simulink library "powerlib"  (Simulink 6.0)
settings: Solver=ode45  SolverMode=SingleTasking  StartTime=0.0  StopTime=10.0  RelTol=1e-3
undefined symbols (not defined in the file or in its folder): com, ctrl1, Da, DiscIntNeverNeededParam, dtha, etat, FA, find_system, Ha, j, Ka, Ki, Kv, q0, Rground, sel, st_a, st_b, st_c, sta, stb, stc, T1, T2, T3, T4
libraries: powerlib_models x30, powerlib x25, simulink_extras x6, powerlib_extras x3, simulink x2
(part 7 of 7)

== system powerlib/Phasor Elements/Static Var Compensator/I1 Time delay  Td ==
  I1 cmplx : Inport  Orientation=left  Port=1  LatchInput=off
  Complex to Real-Imag : ComplexToRealImag  Orientation=left
  Real-Imag to Complex : RealImagToComplex  Orientation=left
  Transport Delay1 : TransportDelay  Orientation=left  DelayTime=Td
  Transport Delay2 : TransportDelay  Orientation=left  DelayTime=Td
  Out1 : Outport  Orientation=left
  wires:
  I1 cmplx/1 -> Complex to Real-Imag/1
  Real-Imag to Complex/1 -> Out1/1
  Complex to Real-Imag/1 -> Transport Delay1/1
  Complex to Real-Imag/2 -> Transport Delay2/1
  Transport Delay1/1 -> Real-Imag to Complex/1
  Transport Delay2/1 -> Real-Imag to Complex/2

== system powerlib/Phasor Elements/Static Var Compensator/I2 Time delay I2 ==
  I1 cmplx : Inport  Orientation=left  Port=1  LatchInput=off
  Complex to Real-Imag : ComplexToRealImag  Orientation=left
  Real-Imag to Complex : RealImagToComplex  Orientation=left
  Transport Delay1 : TransportDelay  Orientation=left  DelayTime=Td
  Transport Delay2 : TransportDelay  Orientation=left  DelayTime=Td
  Out1 : Outport  Orientation=left
  wires:
  Transport Delay2/1 -> Real-Imag to Complex/2
  Transport Delay1/1 -> Real-Imag to Complex/1
  Complex to Real-Imag/2 -> Transport Delay2/1
  Complex to Real-Imag/1 -> Transport Delay1/1
  Real-Imag to Complex/1 -> Out1/1
  I1 cmplx/1 -> Complex to Real-Imag/1

== system powerlib/Phasor Elements/Static Var Compensator/Phasors-->V1 V2 ==
  Vab Vbc cmplx : Inport  Port=1  LatchInput=off
  (a^2)/3 : Gain  Gain=1/3*exp(-j*2*pi/3)  SaturateOnIntegerOverflow=on
  Demux : Demux  Outputs=2
  Gain : Gain  Gain=1/3  SaturateOnIntegerOverflow=on
  Gain1 : Gain  Gain=1/3  SaturateOnIntegerOverflow=on
  Sum3 : Sum  Inputs=+-  SaturateOnIntegerOverflow=on  InputSameDT=on
  Sum4 : Sum  Inputs=+-  SaturateOnIntegerOverflow=on  InputSameDT=on
  V>pu : Gain  Gain=1/Vbase  SaturateOnIntegerOverflow=on
  a/3 : Gain  Gain=1/3*exp(j*2*pi/3)  SaturateOnIntegerOverflow=on
  V1_pu : Outport
  V2_pu : Outport  Port=2
  wires:
  Sum4/1 -> V2_pu/1  "V2"
  (a^2)/3/1 -> Sum3/2
  Demux/2 -> (a^2)/3/1, a/3/1
  Gain/1 -> Sum3/1
  Vab Vbc cmplx/1 -> V>pu/1
  Gain1/1 -> Sum4/1
  a/3/1 -> Sum4/2
  Demux/1 -> Gain/1, Gain1/1
  Sum3/1 -> V1_pu/1  "V1"
  V>pu/1 -> Demux/1

== system powerlib/Phasor Elements/Static Var Compensator/Voltage regulator ==
  V1meas (pu) : Inport  Port=1  LatchInput=off
  Vref (pu) : Inport  Port=2  LatchInput=off
  Break algebraic loop : TransferFcn  Orientation=left  Denominator=[100e-6 1]
  Droop : Gain  Orientation=left  Gain=Xs  SaturateOnIntegerOverflow=on
  Integrator : Integrator  LimitOutput=on  UpperSaturationLimit=Bmax  LowerSaturationLimit=Bmin
  Ki : Gain  Gain=Ki  SaturateOnIntegerOverflow=on
  Kp : Gain  Gain=Kp  SaturateOnIntegerOverflow=on
  Product : Product  Orientation=down  SaturateOnIntegerOverflow=on  InputSameDT=on
  Saturation : Saturate  UpperLimit=Bmax  LowerLimit=Bmin
  Sum : Sum  Inputs=-+-  SaturateOnIntegerOverflow=on  InputSameDT=on
  Sum1 : Sum  SaturateOnIntegerOverflow=on
  B (pu) : Outport  InitialOutput=0
  wires:
  Sum1/1 -> Product/2, B (pu)/1
  Saturation/1 -> Sum1/1
  Integrator/1 -> Sum1/2
  Kp/1 -> Saturation/1
  Product/1 -> Break algebraic loop/1
  Sum/1 -> Kp/1, Ki/1
  Vref (pu)/1 -> Sum/2
  Ki/1 -> Integrator/1
  V1meas (pu)/1 -> Sum/1, Product/1
  Droop/1 -> Sum/3
  Break algebraic loop/1 -> Droop/1

== system powerlib/Power Electronics/Detailed Thyristor/Measurement list ==
  In1 : Inport  Port=1  LatchInput=off
  Bus Creator1 : BusCreator  DialogController=Simulink.DDGSource_Bus  Inputs=2
  Demux : Demux  Outputs=[1,1]
  Out1 : Outport
  wires:
  Demux/2 -> Bus Creator1/2  "Thyristor voltage"
  Demux/1 -> Bus Creator1/1  "Thyristor current"
  Bus Creator1/1 -> Out1/1
  In1/1 -> Demux/1

== system powerlib/Power Electronics/Diode/Measurement list ==
  In1 : Inport  Port=1  LatchInput=off
  Bus Creator1 : BusCreator  DialogController=Simulink.DDGSource_Bus  Inputs=2
  Demux : Demux  Outputs=[1,1]
  Out1 : Outport
  wires:
  In1/1 -> Demux/1
  Bus Creator1/1 -> Out1/1
  Demux/1 -> Bus Creator1/1  "Diode current"
  Demux/2 -> Bus Creator1/2  "Diode voltage"

== system powerlib/Power Electronics/Gto/Measurement list ==
  In1 : Inport  Port=1  LatchInput=off
  Bus Creator1 : BusCreator  DialogController=Simulink.DDGSource_Bus  Inputs=2
  Demux : Demux  Outputs=[1,1]
  Out1 : Outport
  wires:
  Demux/2 -> Bus Creator1/2  "GTO voltage"
  Demux/1 -> Bus Creator1/1  "GTO current"
  Bus Creator1/1 -> Out1/1
  In1/1 -> Demux/1

== system powerlib/Power Electronics/IGBT/Measurement list ==
  In1 : Inport  Port=1  LatchInput=off
  Bus Creator1 : BusCreator  DialogController=Simulink.DDGSource_Bus  Inputs=2
  Demux : Demux  Outputs=[1,1]
  Out1 : Outport
  wires:
  Demux/2 -> Bus Creator1/2  "IGBT voltage"
  Demux/1 -> Bus Creator1/1  "IGBT current"
  Bus Creator1/1 -> Out1/1
  In1/1 -> Demux/1

== system powerlib/Power Electronics/Ideal Switch/Measurement list ==
  In1 : Inport  Port=1  LatchInput=off
  Bus Creator1 : BusCreator  DialogController=Simulink.DDGSource_Bus  Inputs=2
  Demux : Demux  Outputs=[1,1]
  Out1 : Outport
  wires:
  In1/1 -> Demux/1
  Bus Creator1/1 -> Out1/1
  Demux/1 -> Bus Creator1/1  "Switch current"
  Demux/2 -> Bus Creator1/2  "Switch voltage"

== system powerlib/Power Electronics/Mosfet/Measurement list ==
  In1 : Inport  Port=1  LatchInput=off
  Bus Creator1 : BusCreator  DialogController=Simulink.DDGSource_Bus  Inputs=2
  Demux : Demux  Outputs=[1,1]
  Out1 : Outport
  wires:
  In1/1 -> Demux/1
  Bus Creator1/1 -> Out1/1
  Demux/1 -> Bus Creator1/1  "Mosfet current"
  Demux/2 -> Bus Creator1/2  "Mosfet voltage"

== system powerlib/Power Electronics/Thyristor/Measurement list ==
  In1 : Inport  Port=1  LatchInput=off
  Bus Creator1 : BusCreator  DialogController=Simulink.DDGSource_Bus  Inputs=2
  Demux : Demux  Outputs=[1,1]
  Out1 : Outport
  wires:
  In1/1 -> Demux/1
  Bus Creator1/1 -> Out1/1
  Demux/1 -> Bus Creator1/1  "Thyristor current"
  Demux/2 -> Bus Creator1/2  "Thyristor voltage"

== system powerlib/Machines/Steam Turbine and Governor/4 mass shaft/1 mass ==
  Tt_1-4 : Inport  Port=1  LatchInput=off
  dth_gen : Inport  Port=2  LatchInput=off
  Enable : EnablePort
  Ground : Ground
  Ground1 : Ground  Orientation=left
  Mass2 : Subsystem  mask(Generic rotating mass){H=Ha(1), K=Ka(1), D=Da(1), dth0=dtha(1)}
      mask prompts: H "Inertia H (p.u.)"; K "Rigidity K (p.u.):"; D "Damping D (p.u.):"; dth0 "Initial angle deviation delta_theta (rad):"
  Mux : Mux  Inputs=[3 1]
  Mux1 : Mux  Inputs=[3 1]
  Selector : Selector  Elements=sel{1}  InputPortWidth=4
  Terminator : Terminator
  Ts_5-2 : Outport  InitialOutput=[0,0,0,0]
  dw_5-2 : Outport  Port=2  InitialOutput=[0,0,0,0]
  Tm_gen : Outport  Port=3
  wires:
  Mass2/2(Ts_k) -> Tm_gen/1, Mux/2
  dth_gen/1 -> Mass2/3(deltat_k-1)
  Mass2/1(deltat_k) -> Terminator/1
  Ground/1 -> Mass2/1(Ts_k+1)
  Selector/1 -> Mass2/2(Tt_k)
  Mux/1 -> Ts_5-2/1
  Tt_1-4/1 -> Selector/1
  Ground1/1 -> Mux/1, Mux1/1
  Mass2/3(dw) -> Mux1/2
  Mux1/1 -> dw_5-2/1

== system powerlib/Machines/Steam Turbine and Governor/4 mass shaft/2 masses ==
  Tt_1-4 : Inport  Port=1  LatchInput=off
  dth_gen : Inport  Port=2  LatchInput=off
  Enable : EnablePort
  Demux : Demux  Outputs=2
  Ground : Ground
  Ground1 : Ground  Orientation=left
  Mass2 : Subsystem  mask(Generic rotating mass){H=Ha(1), K=Ka(1), D=Da(1), dth0=dtha(1)}
      mask prompts: H "Inertia H (p.u.)"; K "Rigidity K (p.u.):"; D "Damping D (p.u.):"; dth0 "Initial angle deviation delta_theta (rad):"
  Mass3 : Subsystem  mask(Generic rotating mass){H=Ha(2), K=Ka(2), D=Da(2), dth0=dtha(2)}
      mask prompts: H "Inertia H (p.u.)"; K "Rigidity K (p.u.):"; D "Damping D (p.u.):"; dth0 "Initial angle deviation delta_theta (rad):"
  Mux : Mux  Inputs=[ 2 1 1 ]
  Mux1 : Mux  Inputs=[ 2 1 1 ]
  Selector : Selector  Elements=sel{2}  InputPortWidth=4
  Terminator : Terminator
  Ts_5-2 : Outport  InitialOutput=[0,0,0,0]
  dw_5-2 : Outport  Port=2  InitialOutput=[0,0,0,0]
  Tm_gen : Outport  Port=3
  wires:
  Mass2/2(Ts_k) -> Tm_gen/1, Mux/3
  dth_gen/1 -> Mass2/3(deltat_k-1)
  Mass2/1(deltat_k) -> Mass3/3(deltat_k-1)
  Demux/2 -> Mass2/2(Tt_k)
  Ground/1 -> Mass3/1(Ts_k+1)
  Mass3/1(deltat_k) -> Terminator/1
  Mass3/2(Ts_k) -> Mass2/1(Ts_k+1), Mux/2
  Mux/1 -> Ts_5-2/1
  Selector/1 -> Demux/1
  Tt_1-4/1 -> Selector/1
  Demux/1 -> Mass3/2(Tt_k)
  Ground1/1 -> Mux/1, Mux1/1
  Mux1/1 -> dw_5-2/1
  Mass3/3(dw) -> Mux1/2
  Mass2/3(dw) -> Mux1/3

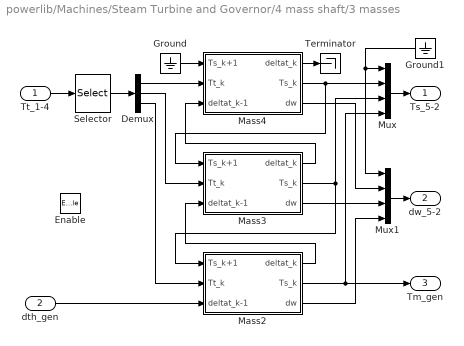
== system powerlib/Machines/Steam Turbine and Governor/4 mass shaft/3 masses ==
  Tt_1-4 : Inport  Port=1  LatchInput=off
  dth_gen : Inport  Port=2  LatchInput=off
  Enable : EnablePort
  Demux : Demux  Outputs=3
  Ground : Ground
  Ground1 : Ground  Orientation=left
  Mass2 : Subsystem  mask(Generic rotating mass){H=Ha(1), K=Ka(1), D=Da(1), dth0=dtha(1)}
      mask prompts: H "Inertia H (p.u.)"; K "Rigidity K (p.u.):"; D "Damping D (p.u.):"; dth0 "Initial angle deviation delta_theta (rad):"
  Mass3 : Subsystem  mask(Generic rotating mass){H=Ha(2), K=Ka(2), D=Da(2), dth0=dtha(2)}
      mask prompts: H "Inertia H (p.u.)"; K "Rigidity K (p.u.):"; D "Damping D (p.u.):"; dth0 "Initial angle deviation delta_theta (rad):"
  Mass4 : Subsystem  mask(Generic rotating mass){H=Ha(3), K=Ka(3), D=Da(3), dth0=dtha(3)}
      mask prompts: H "Inertia H (p.u.)"; K "Rigidity K (p.u.):"; D "Damping D (p.u.):"; dth0 "Initial angle deviation delta_theta (rad):"
  Mux : Mux
  Mux1 : Mux
  Selector : Selector  Elements=sel{3}  InputPortWidth=4
  Terminator : Terminator
  Ts_5-2 : Outport  InitialOutput=[0,0,0,0]
  dw_5-2 : Outport  Port=2  InitialOutput=[0,0,0,0]
  Tm_gen : Outport  Port=3
  wires:
  Mass3/2(Ts_k) -> Mass2/1(Ts_k+1), Mux/3
  Tt_1-4/1 -> Selector/1
  Selector/1 -> Demux/1
  Mass2/2(Ts_k) -> Mux/4, Tm_gen/1
  dth_gen/1 -> Mass2/3(deltat_k-1)
  Mass4/1(deltat_k) -> Terminator/1
  Ground/1 -> Mass4/1(Ts_k+1)
  Demux/1 -> Mass4/2(Tt_k)
  Demux/2 -> Mass3/2(Tt_k)
  Demux/3 -> Mass2/2(Tt_k)
  Mass2/1(deltat_k) -> Mass3/3(deltat_k-1)
  Mass3/1(deltat_k) -> Mass4/3(deltat_k-1)
  Mass4/2(Ts_k) -> Mass3/1(Ts_k+1), Mux/2
  Mass4/3(dw) -> Mux1/2
  Mass3/3(dw) -> Mux1/3
  Mux/1 -> Ts_5-2/1
  Ground1/1 -> Mux/1, Mux1/1
  Mux1/1 -> dw_5-2/1
  Mass2/3(dw) -> Mux1/4

== system powerlib/Machines/Steam Turbine and Governor/4 mass shaft/4 masses ==
  Tt_1-4 : Inport  Port=1  LatchInput=off
  dth_gen : Inport  Port=2  LatchInput=off
  Enable : EnablePort
  Demux : Demux
  Ground : Ground
  Mass2 : Subsystem  mask(Generic rotating mass){H=Ha(1), K=Ka(1), D=Da(1), dth0=dtha(1)}
      mask prompts: H "Inertia H (p.u.)"; K "Rigidity K (p.u.):"; D "Damping D (p.u.):"; dth0 "Initial angle deviation delta_theta (rad):"
  Mass3 : Subsystem  mask(Generic rotating mass){H=Ha(2), K=Ka(2), D=Da(2), dth0=dtha(2)}
      mask prompts: H "Inertia H (p.u.)"; K "Rigidity K (p.u.):"; D "Damping D (p.u.):"; dth0 "Initial angle deviation delta_theta (rad):"
  Mass4 : Subsystem  mask(Generic rotating mass){H=Ha(3), K=Ka(3), D=Da(3), dth0=dtha(3)}
      mask prompts: H "Inertia H (p.u.)"; K "Rigidity K (p.u.):"; D "Damping D (p.u.):"; dth0 "Initial angle deviation delta_theta (rad):"
  Mass5 : Subsystem  mask(Generic rotating mass){H=Ha(4), K=Ka(4), D=Da(4), dth0=dtha(4)}
      mask prompts: H "Inertia H (p.u.)"; K "Rigidity K (p.u.):"; D "Damping D (p.u.):"; dth0 "Initial angle deviation delta_theta (rad):"
  Mux : Mux
  Mux1 : Mux
  Terminator : Terminator
  Ts_5-2 : Outport  InitialOutput=[0,0,0,0]
  dw_5-2 : Outport  Port=2  InitialOutput=[0,0,0,0]
  Tm_gen : Outport  Port=3
  wires:
  Mass2/2(Ts_k) -> Tm_gen/1, Mux/4
  dth_gen/1 -> Mass2/3(deltat_k-1)
  Tt_1-4/1 -> Demux/1
  Mass3/2(Ts_k) -> Mux/3, Mass2/1(Ts_k+1)
  Mass4/2(Ts_k) -> Mux/2, Mass3/1(Ts_k+1)
  Mass5/2(Ts_k) -> Mass4/1(Ts_k+1), Mux/1
  Mass4/1(deltat_k) -> Mass5/3(deltat_k-1)
  Mass3/1(deltat_k) -> Mass4/3(deltat_k-1)
  Mass2/1(deltat_k) -> Mass3/3(deltat_k-1)
  Demux/4 -> Mass2/2(Tt_k)
  Demux/3 -> Mass3/2(Tt_k)
  Demux/2 -> Mass4/2(Tt_k)
  Demux/1 -> Mass5/2(Tt_k)
  Ground/1 -> Mass5/1(Ts_k+1)
  Mass5/1(deltat_k) -> Terminator/1
  Mux/1 -> Ts_5-2/1
  Mass5/3(dw) -> Mux1/1
  Mass4/3(dw) -> Mux1/2
  Mux1/1 -> dw_5-2/1
  Mass3/3(dw) -> Mux1/3
  Mass2/3(dw) -> Mux1/4

== system powerlib/Machines/Steam Turbine and Governor/steam turbine/Stage1 ==
  In1 : Inport  Port=1  LatchInput=off
  Constant1 : Constant  Orientation=down  Value=Ta(4)~=0
  Stage4 : Subsystem  TreatAsAtomicUnit=on
  Switch3 : Switch  Threshold=0.5  InputSameDT=on
  Out1 : Outport
  wires:
  Switch3/1 -> Out1/1
  In1/1 -> Switch3/3, Stage4/1(In1)
  Constant1/1 -> Switch3/2, Stage4/Enable
  Stage4/1(Out1) -> Switch3/1

== system powerlib/Machines/Steam Turbine and Governor/steam turbine/Stage2 ==
  In1 : Inport  Port=1  LatchInput=off
  Constant2 : Constant  Orientation=down  Value=Ta(3)~=0
  Stage3 : Subsystem  TreatAsAtomicUnit=on
  Switch2 : Switch  Threshold=0.5  InputSameDT=on
  Out1 : Outport
  wires:
  In1/1 -> Switch2/3, Stage3/1(In1)
  Switch2/1 -> Out1/1
  Constant2/1 -> Switch2/2, Stage3/Enable
  Stage3/1(Out1) -> Switch2/1

== system powerlib/Machines/Steam Turbine and Governor/steam turbine/Stage3  ==
  In1 : Inport  Port=1  LatchInput=off
  Constant3 : Constant  Orientation=down  Value=Ta(2)~=0
  Stage2 : Subsystem  TreatAsAtomicUnit=on
  Switch1 : Switch  Threshold=0.5  InputSameDT=on
  Out1 : Outport
  wires:
  In1/1 -> Switch1/3, Stage2/1(In1)
  Switch1/1 -> Out1/1
  Constant3/1 -> Switch1/2, Stage2/Enable
  Stage2/1(Out1) -> Switch1/1

== system powerlib/Machines/Steam Turbine and Governor/steam turbine/Stage4 ==
  In1 : Inport  Port=1  LatchInput=off
  Constant4 : Constant  Orientation=down  Value=Ta(1)~=0
  Stage1 : Subsystem  TreatAsAtomicUnit=on
  Switch : Switch  Threshold=0.5  InputSameDT=on
  Out1 : Outport
  wires:
  Switch/1 -> Out1/1
  Stage1/1(Out1) -> Switch/1
  In1/1 -> Switch/3, Stage1/1(In1)
  Constant4/1 -> Switch/2, Stage1/Enable

== system powerlib/Machines/Steam Turbine and Governor/4 mass shaft/1 mass/Mass2 ==
  Ts_k+1 : Inport  Port=1  LatchInput=off
  Tt_k : Inport  Port=2  LatchInput=off
  deltat_k-1 : Inport  Port=3  LatchInput=off
  Gain10 : Gain  Gain=D  SaturateOnIntegerOverflow=on
  Gain11 : Gain  Gain=K  SaturateOnIntegerOverflow=on
  Gain9 : Gain  Gain=1/(2*H)  SaturateOnIntegerOverflow=on
  Integrator6 : Integrator
  Integrator7 : Integrator  InitialCondition=dth0
  Sum11 : Sum  Orientation=left  Inputs=|+-  SaturateOnIntegerOverflow=on  InputSameDT=on
  Sum9 : Sum  Inputs=+|+|-|-  SaturateOnIntegerOverflow=on  InputSameDT=on
  pu2radpersec : Gain  Gain=120*pi  SaturateOnIntegerOverflow=on
  deltat_k : Outport  InitialOutput=0
  Ts_k : Outport  Port=2  InitialOutput=0
  dw : Outport  Port=3  InitialOutput=0
  wires:
  deltat_k-1/1 -> Sum11/2
  Sum11/1 -> Gain11/1
  Integrator7/1 -> deltat_k/1, Sum11/1
  pu2radpersec/1 -> Integrator7/1
  Integrator6/1 -> pu2radpersec/1, Gain10/1, dw/1
  Tt_k/1 -> Sum9/2
  Sum9/1 -> Gain9/1
  Gain10/1 -> Sum9/4
  Gain11/1 -> Ts_k/1, Sum9/3
  Ts_k+1/1 -> Sum9/1
  Gain9/1 -> Integrator6/1

== system powerlib/Machines/Steam Turbine and Governor/4 mass shaft/2 masses/Mass2 ==
  Ts_k+1 : Inport  Port=1  LatchInput=off
  Tt_k : Inport  Port=2  LatchInput=off
  deltat_k-1 : Inport  Port=3  LatchInput=off
  Gain10 : Gain  Gain=D  SaturateOnIntegerOverflow=on
  Gain11 : Gain  Gain=K  SaturateOnIntegerOverflow=on
  Gain9 : Gain  Gain=1/(2*H)  SaturateOnIntegerOverflow=on
  Integrator6 : Integrator
  Integrator7 : Integrator  InitialCondition=dth0
  Sum11 : Sum  Orientation=left  Inputs=|+-  SaturateOnIntegerOverflow=on  InputSameDT=on
  Sum9 : Sum  Inputs=+|+|-|-  SaturateOnIntegerOverflow=on  InputSameDT=on
  pu2radpersec : Gain  Gain=120*pi  SaturateOnIntegerOverflow=on
  deltat_k : Outport  InitialOutput=0
  Ts_k : Outport  Port=2  InitialOutput=0
  dw : Outport  Port=3  InitialOutput=0
  wires:
  deltat_k-1/1 -> Sum11/2
  Sum11/1 -> Gain11/1
  Integrator7/1 -> deltat_k/1, Sum11/1
  pu2radpersec/1 -> Integrator7/1
  Integrator6/1 -> pu2radpersec/1, Gain10/1, dw/1
  Tt_k/1 -> Sum9/2
  Sum9/1 -> Gain9/1
  Gain10/1 -> Sum9/4
  Gain11/1 -> Ts_k/1, Sum9/3
  Ts_k+1/1 -> Sum9/1
  Gain9/1 -> Integrator6/1

== system powerlib/Machines/Steam Turbine and Governor/4 mass shaft/2 masses/Mass3 ==
  Ts_k+1 : Inport  Port=1  LatchInput=off
  Tt_k : Inport  Port=2  LatchInput=off
  deltat_k-1 : Inport  Port=3  LatchInput=off
  Gain10 : Gain  Gain=D  SaturateOnIntegerOverflow=on
  Gain11 : Gain  Gain=K  SaturateOnIntegerOverflow=on
  Gain9 : Gain  Gain=1/(2*H)  SaturateOnIntegerOverflow=on
  Integrator6 : Integrator
  Integrator7 : Integrator  InitialCondition=dth0
  Sum11 : Sum  Orientation=left  Inputs=|+-  SaturateOnIntegerOverflow=on  InputSameDT=on
  Sum9 : Sum  Inputs=+|+|-|-  SaturateOnIntegerOverflow=on  InputSameDT=on
  pu2radpersec : Gain  Gain=120*pi  SaturateOnIntegerOverflow=on
  deltat_k : Outport  InitialOutput=0
  Ts_k : Outport  Port=2  InitialOutput=0
  dw : Outport  Port=3  InitialOutput=0
  wires:
  Ts_k+1/1 -> Sum9/1
  Gain11/1 -> Sum9/3, Ts_k/1
  Gain10/1 -> Sum9/4
  Sum9/1 -> Gain9/1
  Gain9/1 -> Integrator6/1
  Tt_k/1 -> Sum9/2
  Integrator6/1 -> pu2radpersec/1, Gain10/1, dw/1
  pu2radpersec/1 -> Integrator7/1
  Integrator7/1 -> Sum11/1, deltat_k/1
  Sum11/1 -> Gain11/1
  deltat_k-1/1 -> Sum11/2

== system powerlib/Machines/Steam Turbine and Governor/4 mass shaft/3 masses/Mass2 ==
  Ts_k+1 : Inport  Port=1  LatchInput=off
  Tt_k : Inport  Port=2  LatchInput=off
  deltat_k-1 : Inport  Port=3  LatchInput=off
  Gain10 : Gain  Gain=D  SaturateOnIntegerOverflow=on
  Gain11 : Gain  Gain=K  SaturateOnIntegerOverflow=on
  Gain9 : Gain  Gain=1/(2*H)  SaturateOnIntegerOverflow=on
  Integrator6 : Integrator
  Integrator7 : Integrator  InitialCondition=dth0
  Sum11 : Sum  Orientation=left  Inputs=|+-  SaturateOnIntegerOverflow=on  InputSameDT=on
  Sum9 : Sum  Inputs=+|+|-|-  SaturateOnIntegerOverflow=on  InputSameDT=on
  pu2radpersec : Gain  Gain=120*pi  SaturateOnIntegerOverflow=on
  deltat_k : Outport  InitialOutput=0
  Ts_k : Outport  Port=2  InitialOutput=0
  dw : Outport  Port=3  InitialOutput=0
  wires:
  deltat_k-1/1 -> Sum11/2
  Sum11/1 -> Gain11/1
  Integrator7/1 -> deltat_k/1, Sum11/1
  pu2radpersec/1 -> Integrator7/1
  Integrator6/1 -> pu2radpersec/1, Gain10/1, dw/1
  Tt_k/1 -> Sum9/2
  Sum9/1 -> Gain9/1
  Gain10/1 -> Sum9/4
  Gain11/1 -> Ts_k/1, Sum9/3
  Ts_k+1/1 -> Sum9/1
  Gain9/1 -> Integrator6/1

== system powerlib/Machines/Steam Turbine and Governor/4 mass shaft/3 masses/Mass3 ==
  Ts_k+1 : Inport  Port=1  LatchInput=off
  Tt_k : Inport  Port=2  LatchInput=off
  deltat_k-1 : Inport  Port=3  LatchInput=off
  Gain10 : Gain  Gain=D  SaturateOnIntegerOverflow=on
  Gain11 : Gain  Gain=K  SaturateOnIntegerOverflow=on
  Gain9 : Gain  Gain=1/(2*H)  SaturateOnIntegerOverflow=on
  Integrator6 : Integrator
  Integrator7 : Integrator  InitialCondition=dth0
  Sum11 : Sum  Orientation=left  Inputs=|+-  SaturateOnIntegerOverflow=on  InputSameDT=on
  Sum9 : Sum  Inputs=+|+|-|-  SaturateOnIntegerOverflow=on  InputSameDT=on
  pu2radpersec : Gain  Gain=120*pi  SaturateOnIntegerOverflow=on
  deltat_k : Outport  InitialOutput=0
  Ts_k : Outport  Port=2  InitialOutput=0
  dw : Outport  Port=3  InitialOutput=0
  wires:
  Ts_k+1/1 -> Sum9/1
  Gain11/1 -> Sum9/3, Ts_k/1
  Gain10/1 -> Sum9/4
  Sum9/1 -> Gain9/1
  Gain9/1 -> Integrator6/1
  Tt_k/1 -> Sum9/2
  Integrator6/1 -> pu2radpersec/1, Gain10/1, dw/1
  pu2radpersec/1 -> Integrator7/1
  Integrator7/1 -> Sum11/1, deltat_k/1
  Sum11/1 -> Gain11/1
  deltat_k-1/1 -> Sum11/2

== system powerlib/Machines/Steam Turbine and Governor/4 mass shaft/3 masses/Mass4 ==
  Ts_k+1 : Inport  Port=1  LatchInput=off
  Tt_k : Inport  Port=2  LatchInput=off
  deltat_k-1 : Inport  Port=3  LatchInput=off
  Gain10 : Gain  Gain=D  SaturateOnIntegerOverflow=on
  Gain11 : Gain  Gain=K  SaturateOnIntegerOverflow=on
  Gain9 : Gain  Gain=1/(2*H)  SaturateOnIntegerOverflow=on
  Integrator6 : Integrator
  Integrator7 : Integrator  InitialCondition=dth0
  Sum11 : Sum  Orientation=left  Inputs=|+-  SaturateOnIntegerOverflow=on  InputSameDT=on
  Sum9 : Sum  Inputs=+|+|-|-  SaturateOnIntegerOverflow=on  InputSameDT=on
  pu2radpersec : Gain  Gain=120*pi  SaturateOnIntegerOverflow=on
  deltat_k : Outport  InitialOutput=0
  Ts_k : Outport  Port=2  InitialOutput=0
  dw : Outport  Port=3  InitialOutput=0
  wires:
  deltat_k-1/1 -> Sum11/2
  Sum11/1 -> Gain11/1
  Integrator7/1 -> deltat_k/1, Sum11/1
  pu2radpersec/1 -> Integrator7/1
  Integrator6/1 -> pu2radpersec/1, Gain10/1, dw/1
  Tt_k/1 -> Sum9/2
  Gain9/1 -> Integrator6/1
  Sum9/1 -> Gain9/1
  Gain10/1 -> Sum9/4
  Gain11/1 -> Ts_k/1, Sum9/3
  Ts_k+1/1 -> Sum9/1

== system powerlib/Machines/Steam Turbine and Governor/4 mass shaft/4 masses/Mass2 ==
  Ts_k+1 : Inport  Port=1  LatchInput=off
  Tt_k : Inport  Port=2  LatchInput=off
  deltat_k-1 : Inport  Port=3  LatchInput=off
  Gain10 : Gain  Gain=D  SaturateOnIntegerOverflow=on
  Gain11 : Gain  Gain=K  SaturateOnIntegerOverflow=on
  Gain9 : Gain  Gain=1/(2*H)  SaturateOnIntegerOverflow=on
  Integrator6 : Integrator
  Integrator7 : Integrator  InitialCondition=dth0
  Sum11 : Sum  Orientation=left  Inputs=|+-  SaturateOnIntegerOverflow=on  InputSameDT=on
  Sum9 : Sum  Inputs=+|+|-|-  SaturateOnIntegerOverflow=on  InputSameDT=on
  pu2radpersec : Gain  Gain=120*pi  SaturateOnIntegerOverflow=on
  deltat_k : Outport  InitialOutput=0
  Ts_k : Outport  Port=2  InitialOutput=0
  dw : Outport  Port=3  InitialOutput=0
  wires:
  Gain9/1 -> Integrator6/1
  Ts_k+1/1 -> Sum9/1
  Gain11/1 -> Sum9/3, Ts_k/1
  Gain10/1 -> Sum9/4
  Sum9/1 -> Gain9/1
  Tt_k/1 -> Sum9/2
  Integrator6/1 -> pu2radpersec/1, Gain10/1, dw/1
  pu2radpersec/1 -> Integrator7/1
  Integrator7/1 -> Sum11/1, deltat_k/1
  Sum11/1 -> Gain11/1
  deltat_k-1/1 -> Sum11/2

== system powerlib/Machines/Steam Turbine and Governor/4 mass shaft/4 masses/Mass3 ==
  Ts_k+1 : Inport  Port=1  LatchInput=off
  Tt_k : Inport  Port=2  LatchInput=off
  deltat_k-1 : Inport  Port=3  LatchInput=off
  Gain10 : Gain  Gain=D  SaturateOnIntegerOverflow=on
  Gain11 : Gain  Gain=K  SaturateOnIntegerOverflow=on
  Gain9 : Gain  Gain=1/(2*H)  SaturateOnIntegerOverflow=on
  Integrator6 : Integrator
  Integrator7 : Integrator  InitialCondition=dth0
  Sum11 : Sum  Orientation=left  Inputs=|+-  SaturateOnIntegerOverflow=on  InputSameDT=on
  Sum9 : Sum  Inputs=+|+|-|-  SaturateOnIntegerOverflow=on  InputSameDT=on
  pu2radpersec : Gain  Gain=120*pi  SaturateOnIntegerOverflow=on
  deltat_k : Outport  InitialOutput=0
  Ts_k : Outport  Port=2  InitialOutput=0
  dw : Outport  Port=3  InitialOutput=0
  wires:
  deltat_k-1/1 -> Sum11/2
  Sum11/1 -> Gain11/1
  Integrator7/1 -> deltat_k/1, Sum11/1
  pu2radpersec/1 -> Integrator7/1
  Integrator6/1 -> pu2radpersec/1, Gain10/1, dw/1
  Tt_k/1 -> Sum9/2
  Gain9/1 -> Integrator6/1
  Sum9/1 -> Gain9/1
  Gain10/1 -> Sum9/4
  Gain11/1 -> Ts_k/1, Sum9/3
  Ts_k+1/1 -> Sum9/1

== system powerlib/Machines/Steam Turbine and Governor/4 mass shaft/4 masses/Mass4 ==
  Ts_k+1 : Inport  Port=1  LatchInput=off
  Tt_k : Inport  Port=2  LatchInput=off
  deltat_k-1 : Inport  Port=3  LatchInput=off
  Gain10 : Gain  Gain=D  SaturateOnIntegerOverflow=on
  Gain11 : Gain  Gain=K  SaturateOnIntegerOverflow=on
  Gain9 : Gain  Gain=1/(2*H)  SaturateOnIntegerOverflow=on
  Integrator6 : Integrator
  Integrator7 : Integrator  InitialCondition=dth0
  Sum11 : Sum  Orientation=left  Inputs=|+-  SaturateOnIntegerOverflow=on  InputSameDT=on
  Sum9 : Sum  Inputs=+|+|-|-  SaturateOnIntegerOverflow=on  InputSameDT=on
  pu2radpersec : Gain  Gain=120*pi  SaturateOnIntegerOverflow=on
  deltat_k : Outport  InitialOutput=0
  Ts_k : Outport  Port=2  InitialOutput=0
  dw : Outport  Port=3  InitialOutput=0
  wires:
  Ts_k+1/1 -> Sum9/1
  Gain11/1 -> Sum9/3, Ts_k/1
  Gain10/1 -> Sum9/4
  Sum9/1 -> Gain9/1
  Gain9/1 -> Integrator6/1
  Tt_k/1 -> Sum9/2
  Integrator6/1 -> pu2radpersec/1, Gain10/1, dw/1
  pu2radpersec/1 -> Integrator7/1
  Integrator7/1 -> Sum11/1, deltat_k/1
  Sum11/1 -> Gain11/1
  deltat_k-1/1 -> Sum11/2

== system powerlib/Machines/Steam Turbine and Governor/4 mass shaft/4 masses/Mass5 ==
  Ts_k+1 : Inport  Port=1  LatchInput=off
  Tt_k : Inport  Port=2  LatchInput=off
  deltat_k-1 : Inport  Port=3  LatchInput=off
  Gain10 : Gain  Gain=D  SaturateOnIntegerOverflow=on
  Gain11 : Gain  Gain=K  SaturateOnIntegerOverflow=on
  Gain9 : Gain  Gain=1/(2*H)  SaturateOnIntegerOverflow=on
  Integrator6 : Integrator
  Integrator7 : Integrator  InitialCondition=dth0
  Sum11 : Sum  Orientation=left  Inputs=|+-  SaturateOnIntegerOverflow=on  InputSameDT=on
  Sum9 : Sum  Inputs=+|+|-|-  SaturateOnIntegerOverflow=on  InputSameDT=on
  pu2radpersec : Gain  Gain=120*pi  SaturateOnIntegerOverflow=on
  deltat_k : Outport  InitialOutput=0
  Ts_k : Outport  Port=2  InitialOutput=0
  dw : Outport  Port=3  InitialOutput=0
  wires:
  deltat_k-1/1 -> Sum11/2
  Sum11/1 -> Gain11/1
  Integrator7/1 -> deltat_k/1, Sum11/1
  pu2radpersec/1 -> Integrator7/1
  Integrator6/1 -> pu2radpersec/1, Gain10/1, dw/1
  Tt_k/1 -> Sum9/2
  Gain9/1 -> Integrator6/1
  Sum9/1 -> Gain9/1
  Gain10/1 -> Sum9/4
  Gain11/1 -> Ts_k/1, Sum9/3
  Ts_k+1/1 -> Sum9/1

== system powerlib/Machines/Steam Turbine and Governor/steam turbine/Stage1/Stage4 ==
  In1 : Inport  Port=1  LatchInput=off
  Enable : EnablePort
  Transfer Fcn (with initial outputs)3 : simulink_extras/Additional Linear/Transfer Fcn (with initial outputs)  N=[1]  D="[T4  1]"  Y0=f0  U0=f0
  Out1 : Outport  OutputWhenDisabled=reset  InitialOutput=0
  wires:
  In1/1 -> Transfer Fcn (with initial outputs)3/1
  Transfer Fcn (with initial outputs)3/1 -> Out1/1

== system powerlib/Machines/Steam Turbine and Governor/steam turbine/Stage2/Stage3 ==
  In1 : Inport  Port=1  LatchInput=off
  Enable : EnablePort
  Transfer Fcn (with initial outputs)3 : simulink_extras/Additional Linear/Transfer Fcn (with initial outputs)  N=[1]  D="[T3  1]"  Y0=f0  U0=f0
  Out1 : Outport  OutputWhenDisabled=reset  InitialOutput=0
  wires:
  Transfer Fcn (with initial outputs)3/1 -> Out1/1
  In1/1 -> Transfer Fcn (with initial outputs)3/1

== system powerlib/Machines/Steam Turbine and Governor/steam turbine/Stage3 /Stage2 ==
  In1 : Inport  Port=1  LatchInput=off
  Enable : EnablePort
  Transfer Fcn (with initial outputs)3 : simulink_extras/Additional Linear/Transfer Fcn (with initial outputs)  N=[1]  D="[T2  1]"  Y0=f0  U0=f0
  Out1 : Outport  OutputWhenDisabled=reset  InitialOutput=0
  wires:
  In1/1 -> Transfer Fcn (with initial outputs)3/1
  Transfer Fcn (with initial outputs)3/1 -> Out1/1

== system powerlib/Machines/Steam Turbine and Governor/steam turbine/Stage4/Stage1 ==
  In1 : Inport  Port=1  LatchInput=off
  Enable : EnablePort
  Transfer Fcn (with initial outputs)3 : simulink_extras/Additional Linear/Transfer Fcn (with initial outputs)  N=[1]  D="[T1  1]"  Y0=f0  U0=f0
  Out1 : Outport  OutputWhenDisabled=reset  InitialOutput=0
  wires:
  Transfer Fcn (with initial outputs)3/1 -> Out1/1
  In1/1 -> Transfer Fcn (with initial outputs)3/1
